simulink model "TestCompressor"  (R2012b)
settings: Solver=ode45  StartTime=0.0  StopTime=10.0  RelTol=1e-3
settings Model: Creator=tlavelle  LastModifiedBy=tlavelle

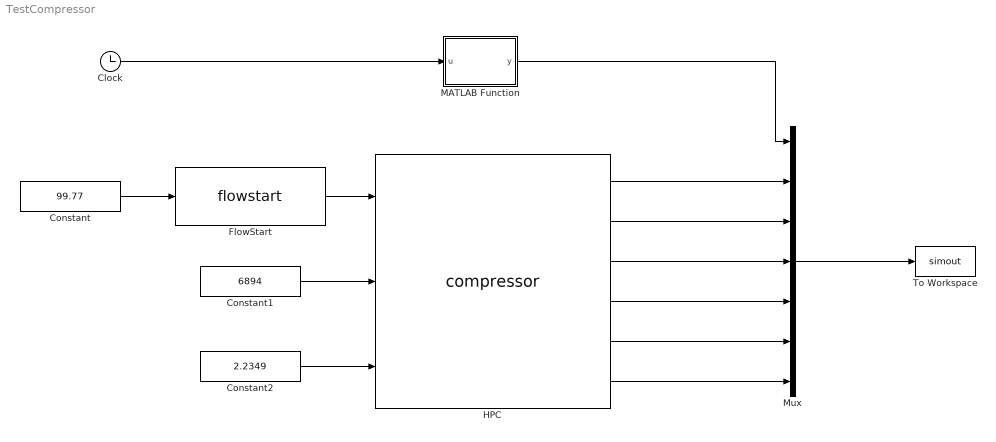
== system TestCompressor ==
  Clock : Clock
  Constant : Constant  Value=99.77
  Constant1 : Constant  Value=6894
  Constant2 : Constant  Value=2.2349
  FlowStart : M-S-Function  FunctionName=flowstart  Parameters=Tt,Pt,comp1,comp2,comp3,comp4,comp5,comp6  mask{Tt=651.82, Pt=21.48, comp1=1, comp2=0, comp3=0, comp4=0, comp5=0, comp6=0}
      mask prompts: Tt "Exit Temperature"; Pt "Exit Pressure"
      mask Display:
      | color('red'); port_label('input',1,'Flow')
      | color('red'); port_label('output',1,'Flow Out')
  HPC : M-S-Function  FunctionName=compressor  Parameters=MapFile,NcDes,effDes,PRdes,RlineDes,Wfrac1,hfrac1,Pfrac1,Wfrac2,hfrac2,Pfrac2,s_eff_in,s_PR_in,s_Wc_in,s_C_Nc_in,IDes  mask{MapFile='HPC.map', NcDes=100, effDes=.8625, PRdes=5.679, RlineDes=2.0805, Wfrac1=.055, hfrac1=1, Pfrac1=1, Wfrac2=.035, hfrac2=1, Pfrac2=1, s_eff_in=1.0137, s_PR_in=.2163, s_Wc_in=.4206, s_C_Nc_in=.0157, IDes=2}
      mask prompts: Wfrac1 "Weight Flow Fraction Bleed1"; hfrac1 "Enthalpy Fraction Bleed 1"; Pfrac1 "Pressure Fraction Bleed 1"; Wfrac2 "Weight Flow Fraction Bleed2"; hfrac2 "Enthalpy Fraction Bleed 2"; Pfrac2 "Pressure Fraction 2"; s_eff_in "Efficiency map scalar"; s_PR_in "Pressure ratio map scalar"; s_Wc_in "Corrected weight flow map scalar"; s_C_Nc_in "Corrected speed map scalar"
      mask Display:
      | color('red'); port_label('input',1,'Flow In')
      | color('yellow'); port_label('input',2,'Speed')
      | color('Blue'); port_label('input',3,'Rline')
      | 
      | color('red'); port_label('output',1,'Flow Out')
      | color('red'); port_label('output',2,'Bleed 1')
      | color('red'); port_label('output',3,'Bleed 2')
      | color('Blue'); port_label('output',4,'Flow Error')
      | color('yellow'); port_label('output',5,'Power')
  MATLAB Function : MATLAB Function  TreatAsAtomicUnit=on
  Mux : Mux  Inputs=7
  To Workspace : ToWorkspace  VariableName=simout  SampleTime=-1  SaveFormat=Timeseries
  wires:
  FlowStart/1 -> HPC/1
  Constant1/1 -> HPC/2
  Constant2/1 -> HPC/3
  Constant/1 -> FlowStart/1
  HPC/1 -> Mux/2
  HPC/2 -> Mux/3
  HPC/3 -> Mux/4
  HPC/4 -> Mux/5
  HPC/5 -> Mux/6
  Clock/1 -> MATLAB Function/1(u)
  HPC/6 -> Mux/7
  MATLAB Function/1(y) -> Mux/1
  Mux/1 -> To Workspace/1

== matlab function TestCompressor/MATLAB Function ==
  data: u input; y output
function y = fcn(u)
%#codegen
eml.extrinsic('set_param');
if u < 3
   set_param('TestCompressor/HPC','IDes','0');
elseif u< 6 
   set_param('TestCompressor/HPC','IDes','1'); 
else 
   set_param('TestCompressor/HPC','IDes','2'); 
end    
y = u;
